simulink model "Reto4Simulink"  (R2018b)
settings: Solver=VariableStepAuto  StartTime=0.0  StopTime=10.0  RelTol=1e-3
libraries: simulink x1
settings Model: Creator=a4lfr  LastModifiedBy=a4lfr

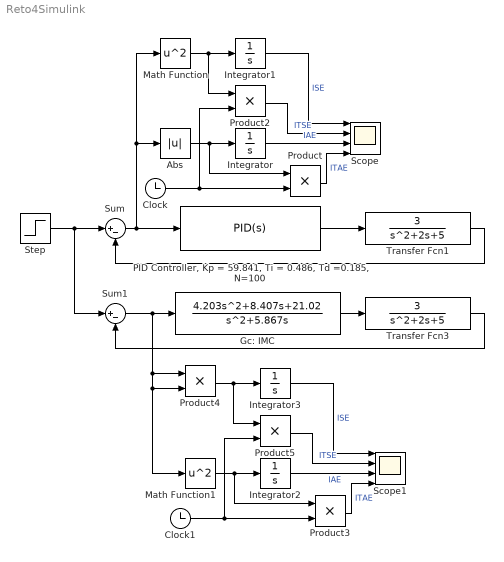
== system Reto4Simulink ==
  Abs : Abs
  Clock : Clock
  Clock1 : Clock
  Gc: IMC : TransferFcn  Numerator=[4.203,8.407,21.02]  Denominator=[1,5.867,0]
  Integrator{,1..3} (4 alike) : Integrator
  Math Function : Math  Operator=square  SaturateOnIntegerOverflow=on
  Math Function1 : Math  Operator=square  SaturateOnIntegerOverflow=on
  "PID Controller, Kp = 59.841, Ti = 0.486, Td =0.185, N=100" : simulink/Continuous/PID Controller  Controller=PID  Form=Ideal  TimeDomain=Continuous-time  SampleTime=-1  IntegratorMethod=Forward Euler  FilterMethod=Forward Euler  ControllerParametersSource=internal  P=59.841  I=1/0.4859  D=0.1847  UseFilter=on  N=100  TunerSelectOption=Transfer Function Based (PID Tuner App)  InitialConditionSource=internal  InitialConditionForIntegrator=0  InitialConditionForFilter=0  DifferentiatorICPrevScaledInput=0  ExternalReset=none  TrackingMode=off  Kt=1  LimitOutput=off  UpperSaturationLimit=inf  LowerSaturationLimit=-inf  LinearizeAsGain=on  AntiWindupMode=none  Kb=1  POutMin=[]  POutMax=[]  IOutMin=[]  IOutMax=[]  DOutMin=[]  DOutMax=[]  NOutMin=[]  NOutMax=[]  SumOutMin=[]  SumOutMax=[]  SaturationOutMin=[]  SaturationOutMax=[]  PParamMin=[]  PParamMax=[]  IParamMin=[]  IParamMax=[]  DParamMin=[]  DParamMax=[]  NParamMin=[]  NParamMax=[]  KbParamMin=[]  KbParamMax=[]  KtParamMin=[]  KtParamMax=[]  KbOutMin=[]  KbOutMax=[]  KtOutMin=[]  KtOutMax=[]  IntegratorOutMin=[]  IntegratorOutMax=[]  FilterOutMin=[]  FilterOutMax=[]  SumI1OutMin=[]  SumI1OutMax=[]  SumI2OutMin=[]  SumI2OutMax=[]  SumI3OutMin=[]  SumI3OutMax=[]  SumI4OutMin=[]  SumI4OutMax=[]  SumDOutMin=[]  SumDOutMax=[]  DifferentiatorOutMin=[]  DifferentiatorOutMax=[]  FilterDiffOutCoefMin=[]  FilterDiffOutCoefMax=[]  ReciprocalOutMin=[]  ReciprocalOutMax=[]  SumDenOutMin=[]  SumDenOutMax=[]  SumNumOutMin=[]  SumNumOutMax=[]  DivideOutMin=[]  DivideOutMax=[]  IntegratorContinuousStateAttributes=''  IntegratorStateMustResolveToSignalObject=off  IntegratorRTWStateStorageClass=Auto  FilterContinuousStateAttributes=''  FilterStateMustResolveToSignalObject=off  FilterRTWStateStorageClass=Auto  ParallelPVariant=Passthrough  IdealPVariant=InternalParameters  IVariant=InternalParameters  DVariant=InternalParameters  IntegratorVariant=Continuous  SatVariant=Disabled  AWVariant=Passthrough  PCopyVariant=Disabled  TRVariant=Disabled  FdbkBlocksVariant=Forward  IdealPFdbkVariant=Disabled  SatFdbkVariant=Disabled  DerivativeFilterVariant=ContFilter  NVariant=InternalParameters  NCopyVariant=Disabled  FilterICVariant=InternalICsFilter  IntegratorICVariant=InternalICs  ExternalResetVariant=Disabled  TRSumVariant=Passthrough  SumFdbkVariant=Disabled  SumVariant=Sum_PID
  Product{,2..5} (5 alike) : Product
  Scope : Scope  NumInputPorts=4
  Scope1 : Scope  NumInputPorts=4
  Step : Step  SampleTime=0
  Sum : Sum  Inputs=|+-
  Sum1 : Sum  Inputs=|+-
  Transfer Fcn1 : TransferFcn  Numerator=[3]  Denominator=[1 2 5]
  Transfer Fcn3 : TransferFcn  Numerator=[3]  Denominator=[1 2 5]
  wires:
  Sum/1 -> "PID Controller, Kp = 59.841, Ti = 0.486, Td =0.185, N=100"/1, Math Function/1, Abs/1
  "PID Controller, Kp = 59.841, Ti = 0.486, Td =0.185, N=100"/1 -> Transfer Fcn1/1
  Transfer Fcn1/1 -> Sum/2
  Transfer Fcn3/1 -> Sum1/2
  Step/1 -> Sum1/1, Sum/1
  Gc: IMC/1 -> Transfer Fcn3/1
  Abs/1 -> Integrator/1, Product/1
  Clock/1 -> Product/2, Product2/2
  Integrator/1 -> Scope/3  "IAE"
  Product/1 -> Scope/4  "ITAE"
  Math Function/1 -> Integrator1/1, Product2/1
  Integrator1/1 -> Scope/1  "ISE"
  Product2/1 -> Scope/2  "ITSE"
  Math Function1/1 -> Integrator2/1, Product3/1
  Sum1/1 -> Product4/1, Math Function1/1, Product4/2, Gc: IMC/1
  Product4/1 -> Integrator3/1, Product5/1
  Product3/1 -> Scope1/4  "ITAE"
  Integrator2/1 -> Scope1/3  "IAE"
  Integrator3/1 -> Scope1/1  "ISE"
  Clock1/1 -> Product3/2, Product5/2
  Product5/1 -> Scope1/2  "ITSE"
